simulink model "mpc_halo"  (R2019b)
settings: Solver=ode45  StartTime=0.0  StopTime=simTime  MaxStep=0.01  RelTol=1e-3  EnableMultiTasking=on
values from neighbouring files (symbols this model uses):
  a = zeros(2,1)    [init.m]    (also in init_halo_casadi.m)
  b = zeros(2,1)    [init.m]    (also in init_halo_casadi.m)
  delta = 0.1    [init.m]
  disturbance = 1    [init.m]
  Gsc = 1360.8    [init.m]    (also in init_halo_casadi.m)
  mu = 0.012149    [casadi_block.m]    (also in init.m; init_halo_casadi.m)
  phi = 0    [init.m]    (also in init_halo_casadi.m)
  sped = 300000    [init.m]    (also in init_halo_casadi.m)
  srp = 1    [init.m]
  x0 = [1;0;0;0;0;0]    [init.m]    (also in init_halo_casadi.m = full(st))
  zeta = 0.9252    [init.m]    (also in init_halo_casadi.m)
settings Model: Creator=jgillis  LastModifiedBy=mohd-
settings DataIOCC: LimitDataPoints=on  SaveFormat=Array  ReturnWorkspaceOutputs=off
settings OptimizationCC: LifeSpan=inf
settings DebuggingCC: SolverPrmCheckMsg=warning  SFUnexpectedBacktrackingDiag=warning  SFNoUnconditionalDefaultTransitionDiag=warning  SFExecutionAtInitializationDiag=none  ArithmeticOperatorsInVariantConditions=warning
settings HardwareCC: ProdBitPerPointer=32  ProdBitPerSizeT=32  ProdBitPerPtrDiffT=32  ProdLargestAtomicFloat=None  ProdIntDivRoundTo=Undefined  ProdEndianess=Unspecified  ProdWordSize=32  ProdHWDeviceType=32-bit Generic
settings ModelReferenceCC: PropagateSignalLabelsOutOfModel=off
settings SFSimCC: SimUseLocalCustomCode=off  CustomCodeUndefinedFunction=UseInterfaceOnly
settings RTWCC: RTWUseLocalCustomCode=off
settings CodeAppCC: StateflowObjectComments=on
settings GRTTargetCC: TargetLangStandard=C89/C90 (ANSI)  GeneratePreprocessorConditionals=Disable all
settings ConfigComp: CovMetricSettings=dw  CovHtmlReporting=on  CovSaveCumulativeToWorkspaceVar=on  CovSaveSingleToWorkspaceVar=on  CovExternalEMLEnable=off  CovSFcnEnable=off

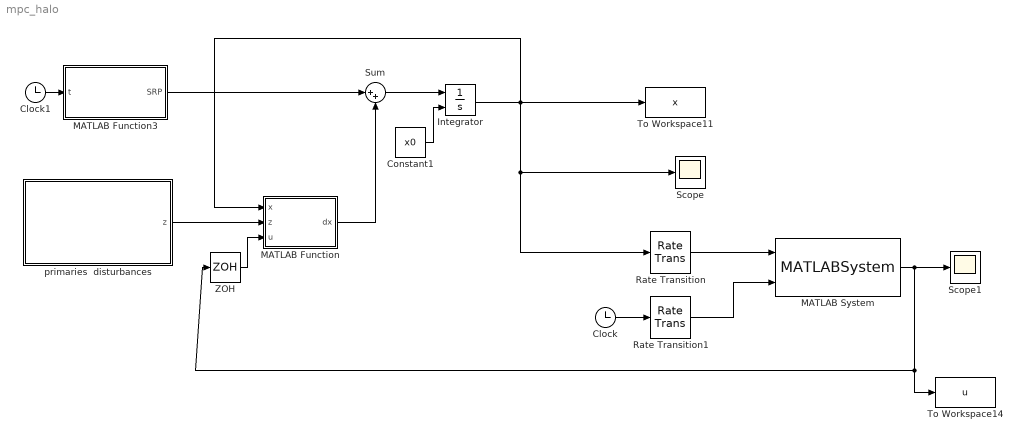
== system mpc_halo ==
  Clock : Clock
  Clock1 : Clock
  Constant1 : Constant  Value=x0
  Integrator : Integrator  InitialConditionSource=external  InitialCondition=[1 0]'
  MATLAB Function : MATLAB Function  TreatAsAtomicUnit=on
  MATLAB Function3 : MATLAB Function  TreatAsAtomicUnit=on
  MATLAB System : MATLABSystem  System=casadi_block  SimulateUsing=Interpreted execution
      mask Type: casadi_block
      mask Display:
      | disp('casadi_block');
      | port_label('input',1,'x');
      | port_label('input',2,'t');
      | port_label('output',1,'u');
  Rate Transition : RateTransition  OutPortSampleTime=delta
  Rate Transition1 : RateTransition  OutPortSampleTime=delta
  Scope : Scope
  Scope1 : Scope
  Sum : Sum  Inputs=|++
  To Workspace11 : ToWorkspace  VariableName=x  SampleTime=10^-3
      settings: Save2DSignal=2-D array (concatenate along first dimension)
  To Workspace14 : ToWorkspace  VariableName=u  SampleTime=10^-3
      settings: Save2DSignal=2-D array (concatenate along first dimension)
  ZOH : ZeroOrderHold  SampleTime=delta
  primaries  disturbances : Subsystem
  wires:
  MATLAB Function/1(dx) -> Sum/2
  Integrator/1 -> Rate Transition/1, Scope/1, To Workspace11/1, MATLAB Function/1(x)
  Constant1/1 -> Integrator/2
  MATLAB System/1 -> Scope1/1, ZOH/1, To Workspace14/1
  ZOH/1 -> MATLAB Function/3(u)
  Clock/1 -> Rate Transition1/1
  Rate Transition/1 -> MATLAB System/1
  Rate Transition1/1 -> MATLAB System/2
  Sum/1 -> Integrator/1
  primaries  disturbances/1(z) -> MATLAB Function/2(z)
  Clock1/1 -> MATLAB Function3/1(t)
  MATLAB Function3/1(SRP) -> Sum/1

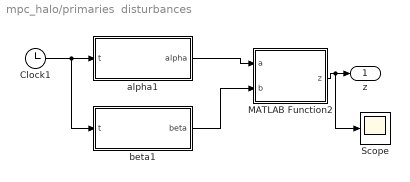
== system mpc_halo/primaries  disturbances ==
  Clock1 : Clock
  MATLAB Function2 : MATLAB Function  TreatAsAtomicUnit=on
  Scope : Scope
  alpha1 : MATLAB Function  TreatAsAtomicUnit=on
  beta1 : MATLAB Function  TreatAsAtomicUnit=on
  z : Outport
  wires:
  Clock1/1 -> beta1/1(t), alpha1/1(t)
  beta1/1(beta) -> MATLAB Function2/2(b)
  alpha1/1(alpha) -> MATLAB Function2/1(a)
  MATLAB Function2/1(z) -> Scope/1, z/1

== matlab function mpc_halo/MATLAB Function3 ==
  data: SRP output; srp parameter; Gsc parameter; sped parameter; zeta parameter; t input
function SRP = fcn(srp, Gsc, sped, zeta,t)

if srp == 1
    SRP = [zeros(3,1);(Gsc/sped)*(cos(zeta*t))^2;(Gsc/sped)*(sin(zeta*t))^2;0];
else
    SRP = zeros(6,1);
end

== matlab function mpc_halo/MATLAB Function ==
  data: x input; z input; u input; dx output; mu parameter
function dx = rhs(x,z, u, mu)
%#codegen

x1 = x(1:3);
x2 = x(4:6);
M = [-1 0 0;
    0 -1 0;
    0 0 0];

N = [0 -1 0;
    1 0 0;
    0 0 0];

d1r = [-mu - z(4)/(1-mu);0;0];
d2r = [1-mu + z(4)/mu;0;0];

ed1 = x1 - d1r;
absed1 = sqrt(ed1(1)^2+ed1(2)^2+ed1(3)^2);
ed2 = x1 - d2r;
absed2 = sqrt(ed2(1)^2+ed2(2)^2+ed2(3)^2);

f1 = x2;
f2 = -M*x1 - 2*N*x2 - (2*M*x1 + 2*N*x2)*z(1) ...
           - M*x1*z(2) - N*x1*z(3) - ed1*(1 - mu)/absed1^3 ...
           - ed2*mu/absed2^3;
F = [f1; f2];
G = [zeros(3); eye(3)];


dx = F + G*u;

end

== matlab function mpc_halo/primaries  disturbances/MATLAB Function2 ==
  data: a input; z output; b input; mu parameter; disturbance parameter
function z = z(a,b,mu, disturbance)
%#codegen
if disturbance == 1
    z = [b;mu*(1-mu)*a];
else
    z = zeros(4,1);
end

== matlab function mpc_halo/primaries  disturbances/alpha1 ==
  data: t input; alpha output; a parameter; phi parameter; e parameter
function alpha = a(t,a,phi,e)
%#codegen

a1 = a(1)*e*cos(t+phi);
alpha = a1;

== matlab function mpc_halo/primaries  disturbances/beta1 ==
  data: t input; beta output; b parameter; phi parameter; e parameter
function beta = b(t,b,phi,e)
%#codegen
b1 = b(1)*e*cos(t+phi);
bd = -b(1)*e*sin(t+phi);
beta = [b1;0;bd];
